simulink model "osservatoreDinamicoSistemaNonLineare"  (R2023b)
settings: Solver=VariableStepAuto  StartTime=0.0  StopTime=10.0  RelTol=1e-3
values from neighbouring files (symbols this model uses):
  AL = A-L*C    [ScriptProgetto.m]
  b = 0.25    [ScriptProgetto.m]
  BL = [B L]    [ScriptProgetto.m]
  CL = eye(3)    [ScriptProgetto.m]
  DL = zeros(3, 2)    [ScriptProgetto.m]
  g = 9.81    [ScriptProgetto.m]
  K = 0.5    [ScriptProgetto.m]
  Ka = acker(A, B, [-1 -2 -4.95/2])    [ScriptProgetto.m]
  M = 3059100    [ScriptProgetto.m]
  meq = rhoa*v - M    (= 6210900)    [ScriptProgetto.m]
  rhoa = 1000    [ScriptProgetto.m]
  v = 9270    [ScriptProgetto.m]
  x1eq = heq    (= 0)    [ScriptProgetto.m]
  x2eq = 0    [ScriptProgetto.m]
  x3eq = meq    (= 6210900)    [ScriptProgetto.m]
undefined symbols (not defined in the file or in its folder): ueq, yeq
settings Model: Creator=angel  LastModifiedBy=martinhaugen
settings SolverCC: AlgebraicLoopSolver=TrustRegion
settings DataIOCC: ReturnWorkspaceOutputs=off
settings DebuggingCC: UnconnectedInputMsg=warning  UnconnectedOutputMsg=warning  UnconnectedLineMsg=warning  ArithmeticOperatorsInVariantConditions=warning
settings ModelReferenceCC: EnableRefExpFcnMdlSchedulingChecks=on
settings SFSimCC: SimUseLocalCustomCode=off  CustomCodeUndefinedFunction=UseInterfaceOnly
settings RTWCC: RTWUseLocalCustomCode=off
settings CodeAppCC: StateflowObjectComments=on

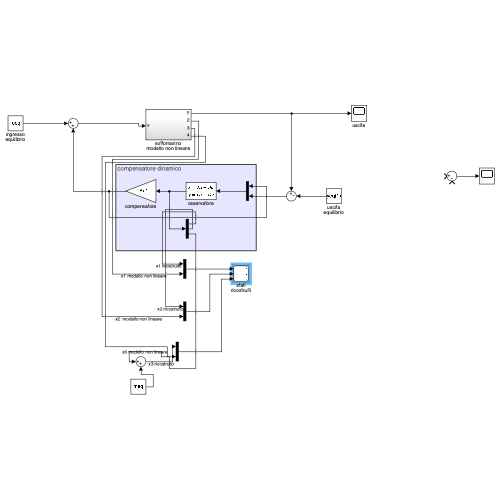
[thumbnail: Simulink's stored preview of the top-level diagram]
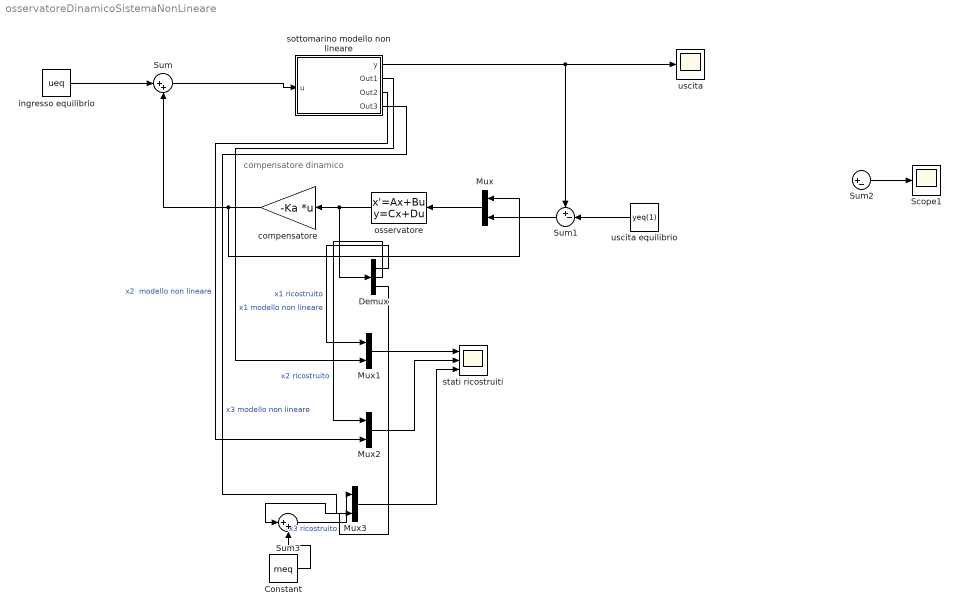
== system osservatoreDinamicoSistemaNonLineare ==
  note: compensatore dinamico
  Constant : Constant  Value=meq
  Demux : Demux  Outputs=3
  Mux{,1..3} (4 alike) : Mux  Inputs=2
  Scope1 : Scope
  Sum : Sum  Inputs=|++
  Sum1 : Sum  Inputs=+-|
  Sum2 : Sum  Inputs=|+-
  Sum3 : Sum  Inputs=|++
  compensatore : Gain  Gain=-Ka  Multiplication=Matrix(K*u)
  ingresso equilibrio : Constant  Value=ueq
  osservatore : StateSpace  A=AL  B=BL  C=CL  D=DL  InitialCondition=[0; 0; 0]
  sottomarino modello non lineare : Subsystem
  stati ricostruiti : Scope  NumInputPorts=3
  uscita : Scope
  uscita equilibrio : Constant  Value=yeq(1)
  wires:
  ingresso equilibrio/1 -> Sum/1
  osservatore/1 -> Demux/1, compensatore/1
  sottomarino modello non lineare/1(y) -> Sum1/1, uscita/1
  Sum/1 -> sottomarino modello non lineare/1(u)
  compensatore/1 -> Mux/1, Sum/2
  uscita equilibrio/1 -> Sum1/2
  Mux/1 -> osservatore/1
  Sum1/1 -> Mux/2
  Sum2/1 -> Scope1/1
  Mux1/1 -> stati ricostruiti/1
  Mux2/1 -> stati ricostruiti/2
  Mux3/1 -> stati ricostruiti/3
  Demux/1 -> Mux1/1  "x1 ricostruito"
  sottomarino modello non lineare/2(Out1) -> Mux1/2  "x1 modello non lineare"
  sottomarino modello non lineare/3(Out2) -> Mux2/2  "x2  modello non lineare"
  Demux/2 -> Mux2/1  "x2 ricostruito"
  sottomarino modello non lineare/4(Out3) -> Mux3/2  "x3 modello non lineare"
  Demux/3 -> Sum3/1
  Constant/1 -> Sum3/2
  Sum3/1 -> Mux3/1  "x3 ricostruito"

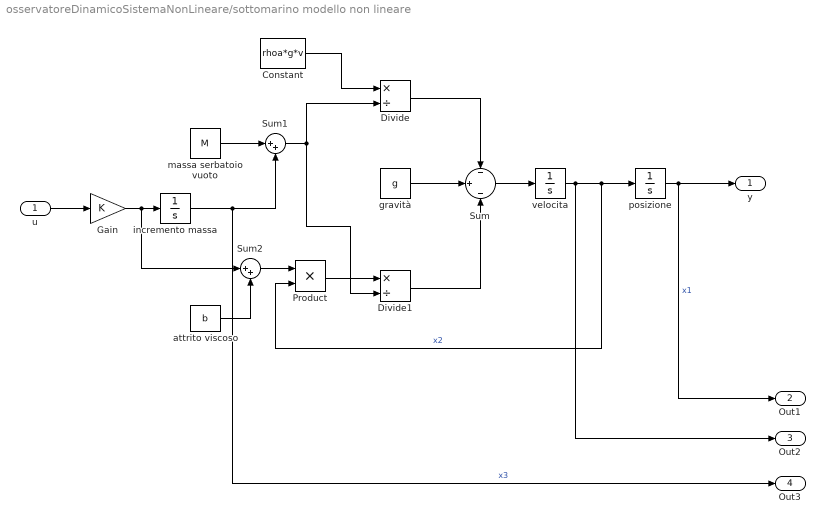
== system osservatoreDinamicoSistemaNonLineare/sottomarino modello non lineare ==
  u : Inport
  Constant : Constant  Value=rhoa*g*v
  Divide : Product  Inputs=*/
  Divide1 : Product  Inputs=*/
  Gain : Gain  Gain=K
  Product : Product
  Sum : Sum  Inputs=-|+|-
  Sum1 : Sum  Inputs=|++
  Sum2 : Sum  Inputs=|++
  attrito viscoso : Constant  Value=b
  gravità : Constant  Value=g
  incremento massa : Integrator  InitialCondition=x3eq
  massa serbatoio vuoto : Constant  Value=M
  posizione : Integrator  InitialCondition=x1eq - 0.4
  velocita : Integrator  InitialCondition=x2eq
  y : Outport
  Out1 : Outport  Port=2
  Out2 : Outport  Port=3
  Out3 : Outport  Port=4
  wires:
  incremento massa/1 -> Out3/1, Sum1/2  "x3"
  Sum1/1 -> Divide/2, Divide1/2
  gravità/1 -> Sum/2
  Constant/1 -> Divide/1
  posizione/1 -> Out1/1, y/1  "x1"
  massa serbatoio vuoto/1 -> Sum1/1
  Sum2/1 -> Product/1
  u/1 -> Gain/1
  Product/1 -> Divide1/1
  velocita/1 -> Out2/1, posizione/1, Product/2  "x2"
  Divide/1 -> Sum/1
  attrito viscoso/1 -> Sum2/2
  Sum/1 -> velocita/1
  Gain/1 -> Sum2/1, incremento massa/1
  Divide1/1 -> Sum/3
